simulink model "staticbalance"  (R2013b)
settings: Solver=ode45  StartTime=0.0  StopTime=50  FixedStep=0.0004  RelTol=1e-3
values from neighbouring files (symbols this model uses):
  K = [2*k -1*k;-1*k 2*k]    [q1_assignment.m]    (also in q2.m = [10 -1;-1 10]; q2_assignment.m = [10 -1;-1 10])
  phi = 2*t*pi    [john (1).m]
  r = 2    [john (1).m]    (also in q2.m = [r1;r2])
  w = sqrt(diag(lam))    [q2.m]
  z = 0.395    [cep.m]    (also in john (1).m = 5; vib.m = (c/m)/(2*wn))
undefined symbols (not defined in the file or in its folder): m_b, m_s, r_b
settings Model: Creator=Zeerak Nadeem Wyne  LastModifiedBy=Zeerak Nadeem Wyne

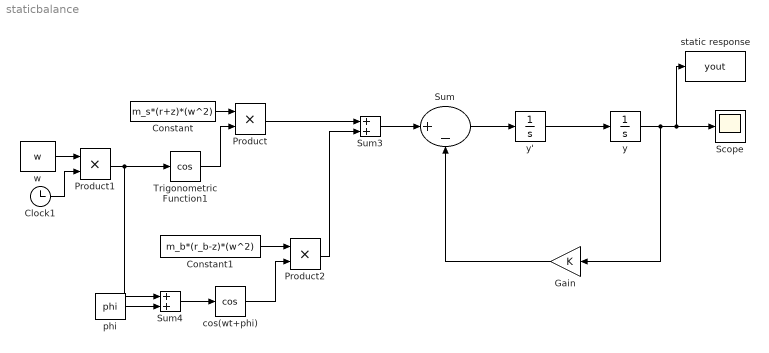
== system staticbalance ==
  Clock1 : Clock
  Constant : Constant  Value=m_s*(r+z)*(w^2)
  Constant1 : Constant  Value=m_b*(r_b-z)*(w^2)
  Gain : Gain  Gain=K
  Product : Product
  Product1 : Product
  Product2 : Product
  Scope : Scope
  Sum : Sum  Inputs=|+-
  Sum3 : Sum
  Sum4 : Sum
  Trigonometric Function1 : Trigonometry  Operator=cos
  "cos(wt+phi) " : Trigonometry  Operator=cos
  "phi " : Constant  Value=phi
  static response : ToWorkspace  VariableName=yout  SampleTime=-1
  "w " : Constant  Value=w
  "y " : Integrator
  y' : Integrator
  wires:
  Sum3/1 -> Sum/1
  Sum/1 -> y'/1
  y'/1 -> "y "/1
  "y "/1 -> Gain/1, static response/1, Scope/1
  Gain/1 -> Sum/2
  Clock1/1 -> Product1/2
  "w "/1 -> Product1/1
  Trigonometric Function1/1 -> Product/2
  Constant/1 -> Product/1
  Product/1 -> Sum3/1
  "cos(wt+phi) "/1 -> Product2/2
  Constant1/1 -> Product2/1
  Product2/1 -> Sum3/2
  Product1/1 -> Sum4/1, Trigonometric Function1/1
  "phi "/1 -> Sum4/2
  Sum4/1 -> "cos(wt+phi) "/1
